simulink model "parrot_host"  (R2024a)
settings: Solver=FixedStepDiscrete  StartTime=0  StopTime=10  RelTol=1e-3
undefined symbols (not defined in the file or in its folder): f
libraries: instrumentlib x1
settings Model: ExtModeTrigDuration=80  Creator=The MathWorks, Inc.  LastModifiedBy=puian
settings SolverCC: AlgebraicLoopSolver=TrustRegion
settings OptimizationCC: DefaultParameterBehavior=Inlined  EnhancedBackFolding=on  PassReuseOutputArgsAs=Individual arguments  MaxStackSize=64  OptimizeBlockOrder=speed  DifferentSizesBufferReuse=on  OptimizationCustomize=off  EfficientTunableParamExpr=on
settings DebuggingCC: ParameterTunabilityLossMsg=error  UnconnectedInputMsg=warning  UnconnectedOutputMsg=warning  UnconnectedLineMsg=warning  ArithmeticOperatorsInVariantConditions=warning
settings HardwareCC: ProdBitPerPointer=32  ProdBitPerSizeT=32  ProdBitPerPtrDiffT=32  ProdLargestAtomicInteger=Long  ProdWordSize=32  ProdHWDeviceType=ARM Compatible->ARM 9  UseEmbeddedCoderFeatures=off  UseSimulinkCoderFeatures=off
settings ModelReferenceCC: EnableRefExpFcnMdlSchedulingChecks=on
settings SFSimCC: SimUseLocalCustomCode=off  MATLABDynamicMemAlloc=off  CustomCodeUndefinedFunction=UseInterfaceOnly
settings RTWCC: Description=Embedded Coder  SystemTargetFile=ert.tlc  TemplateMakefile=ert_default_tmf  GenerateReport=on  RTWUseLocalCustomCode=off  Toolchain=Sourcery G++ Lite GNU Toolchain for Drones  IncludeHyperlinkInReport=on  LaunchReport=on  GenerateTraceInfo=on  GenerateTraceReport=on  GenerateTraceReportSl=on  GenerateTraceReportSf=on  GenerateTraceReportEml=on  GPUComputeCapability=3.5
settings CodeAppCC: ForceParamTrailComments=on  IgnoreCustomStorageClasses=off  OperatorAnnotations=on  SimulinkDataObjDesc=on  SFDataObjDesc=on  InsertBlockDesc=on
settings ERTTargetCC: InlinedParameterPlacement=NonHierarchical  ERTCustomFileTemplate=example_file_process.tlc

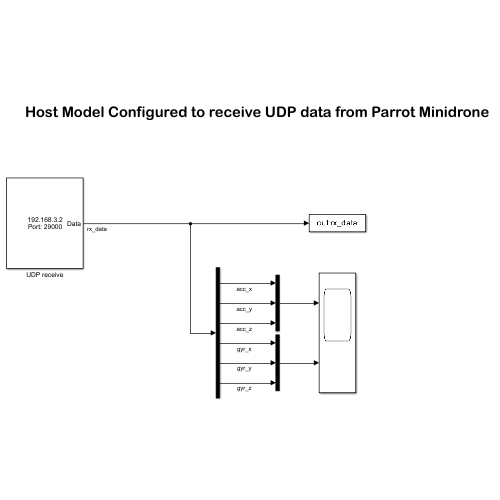
[thumbnail: Simulink's stored preview of the top-level diagram]
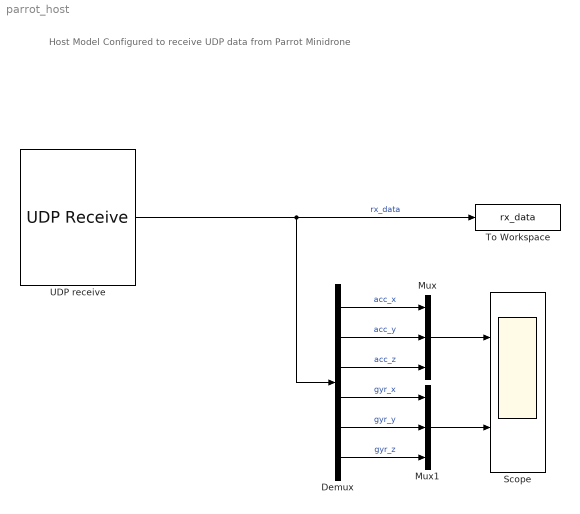
== system parrot_host ==
  note: Host Model Configured to receive UDP data from Parrot Minidrone
  Demux : Demux  Outputs=6
  Mux : Mux  Inputs=3
  Mux1 : Mux  Inputs=3
  Scope : Scope  NumInputPorts=2
  To Workspace : ToWorkspace  VariableName=rx_data  SaveFormat=Structure With Time  SampleTime=-1
  UDP receive : instrumentlib/UDP Receive  LocalAddress=192.168.3.2  LocalPort=29000  EnablePortSharing=off  Host=192.168.3.1  Port=29000  GetLatestData=on  DataSize=6  DataType=single  ASCIIFormatting=%f,  Terminator=LF  CustomTerminator=10  ByteOrder=little-endian  EnableBlockingMode=on  Timeout=10  SampleTime=0.02  SimulateUsing=Interpreted execution
  wires:
  Demux/3 -> Mux/3  "acc_z"
  UDP receive/1 -> To Workspace/1, Demux/1  "rx_data"
  Demux/2 -> Mux/2  "acc_y"
  Demux/6 -> Mux1/3  "gyr_z"
  Mux/1 -> Scope/1
  Demux/5 -> Mux1/2  "gyr_y"
  Demux/4 -> Mux1/1  "gyr_x"
  Mux1/1 -> Scope/2
  Demux/1 -> Mux/1  "acc_x"
